simulink model "generate_joint_position_motion"  (R2023a)
settings: Solver=FixedStepDiscrete  StartTime=0.0  StopTime=inf  FixedStep=0.001  RelTol=1e-3  EnableMultiTasking=on
PreLoadFcn:
  | frs = FrankaRobotSettings;
libraries: franka_simulink_library x5
settings Model: SimulationMode=external  ExtModeTrigDuration=10000  Creator=vasi_ko  LastModifiedBy=kvasios
settings SolverCC: AlgebraicLoopSolver=TrustRegion
settings DataIOCC: LimitDataPoints=on  SaveFormat=Array  ReturnWorkspaceOutputs=off
settings OptimizationCC: DefaultParameterBehavior=Inlined  EnhancedBackFolding=on  PassReuseOutputArgsThreshold=0  OptimizeBlockOrder=speed  DifferentSizesBufferReuse=on  OptimizationCustomize=off
settings DebuggingCC: SolverPrmCheckMsg=warning  ParameterTunabilityLossMsg=error  UnconnectedInputMsg=warning  UnconnectedOutputMsg=warning  UnconnectedLineMsg=warning  SFUnexpectedBacktrackingDiag=warning  SFNoUnconditionalDefaultTransitionDiag=warning  SFExecutionAtInitializationDiag=none  ArithmeticOperatorsInVariantConditions=warning
settings ModelReferenceCC: EnableRefExpFcnMdlSchedulingChecks=on  PropagateSignalLabelsOutOfModel=off
settings SFSimCC: SimUseLocalCustomCode=off  MATLABDynamicMemAlloc=off  CustomCodeUndefinedFunction=UseInterfaceOnly  SimTargetLang=C++
settings RTWCC: RTWVerbose=off  RTWUseLocalCustomCode=off  BuildConfiguration=Faster Runs  TargetLang=C++  DLArmComputeVersion=19.05
settings CodeAppCC: ForceParamTrailComments=on  OperatorAnnotations=on
settings ConfigComp: CovMetricSettings=dw  CovSaveCumulativeToWorkspaceVar=on  CovSaveSingleToWorkspaceVar=on  CovExternalEMLEnable=off  CovSFcnEnable=off

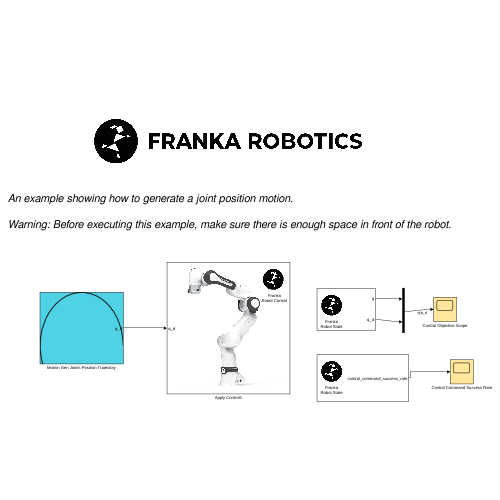
[thumbnail: Simulink's stored preview of the top-level diagram]
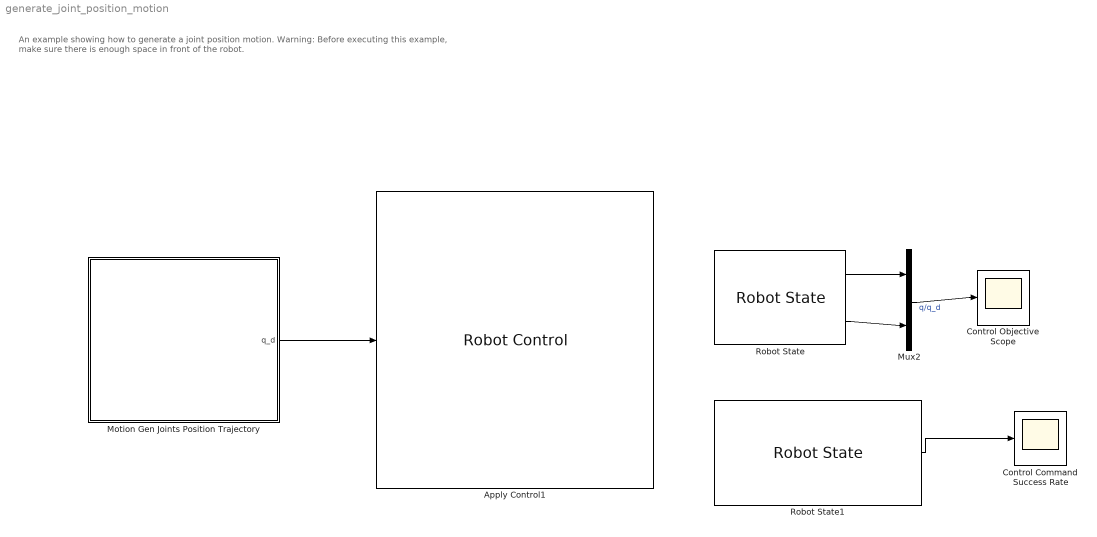
== system generate_joint_position_motion ==
  note: An example showing how to generate a joint position motion.
      |
      | Warning: Before executing this example, make sure there is enough space in front of the robot.
  Apply Control1 : franka_simulink_library/Robot Control  robot_ip=frs.robot_ip  gripper_selection=None  control_mode=Joint Positions - Internal Controller Mode  controller_choice=Joint Impedance Controller  joint_impedance=frs.joint_impedance_stiffness  cartesian_impedance=[3000, 3000, 3000, 300, 300, 300]  rate_limiter=on  cuttoff_frequency=frs.cutoff_frequency  elbow_control=off  collision_thresholds=frs.collision_thresholds.getAs1DArray  load_inertia=frs.load_inertia.getAs1DArray  NE_T_EE=frs.NE_T_EE(:)  EE_T_K=frs.EE_T_K(:)  init_joint_configuration_req=on  init_joint_configuration=frs.home_configuration
      settings: SourceProductName=Franka Robotics Simulink Support Package
  Control Command Success Rate : Scope
  Control Objective Scope : Scope
  Motion Gen Joints Position Trajectory : Subsystem
      mask Display:
      | pos = get_param(gcb, 'Position');
      | width = pos(3) - pos(1);
      | x = [0:width];
      | y = sin(x/180*pi);
      | % Parameters 'm' and 'b' must be defined in 'Parameters & Dialog' pane.
      | plot(cos(x/180*pi), sin(x/180*pi));
      | 
      | port_label('output',1,'q_d');
  Mux2 : Mux  Inputs=2
  Robot State : franka_simulink_library/Robot State  robot_ip=frs.robot_ip  signals_requested='q q_d'
      settings: SourceProductName=Franka Robotics Simulink Support Package
  Robot State1 : franka_simulink_library/Robot State  robot_ip=frs.robot_ip  signals_requested='control_command_success_rate'
      settings: SourceProductName=Franka Robotics Simulink Support Package
  wires:
  Robot State/2 -> Mux2/2
  Mux2/1 -> Control Objective Scope/1  "q/q_d"
  Motion Gen Joints Position Trajectory/1(q_d) -> Apply Control1/1
  Robot State/1 -> Mux2/1
  Robot State1/1 -> Control Command Success Rate/1

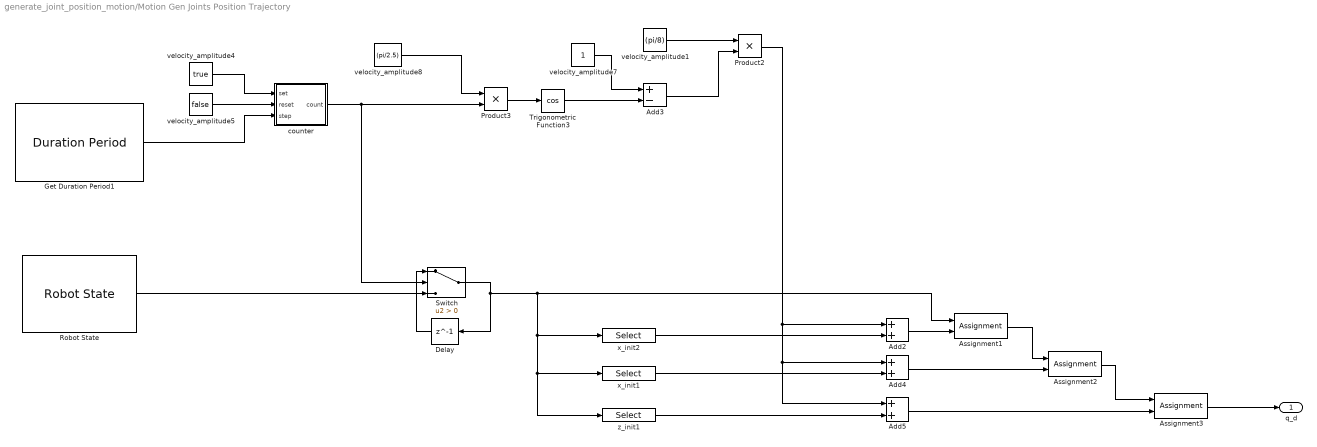
== system generate_joint_position_motion/Motion Gen Joints Position Trajectory ==
  Add2 : Sum
  Add3 : Sum  Inputs=+-
  Add4 : Sum
  Add5 : Sum
  Assignment1 : Assignment  DiagnosticForDimensions=Warning  IndexOptions=Index vector (dialog)  Indices=4  OutputSizes=1
  Assignment2 : Assignment  DiagnosticForDimensions=Warning  IndexOptions=Index vector (dialog)  Indices=5  OutputSizes=1
  Assignment3 : Assignment  DiagnosticForDimensions=Warning  IndexOptions=Index vector (dialog)  Indices=7  OutputSizes=1
  Delay : Delay  DelayLength=1
  Get Duration Period1 : franka_simulink_library/Duration Period  robot_ip=frs.robot_ip
      settings: SourceProductName=Franka Robotics Simulink Support Package
  Product2 : Product
  Product3 : Product
  Robot State : franka_simulink_library/Robot State  robot_ip=frs.robot_ip  signals_requested='q_d'
      settings: SourceProductName=Franka Robotics Simulink Support Package
  Switch : Switch  Criteria=u2 > Threshold  SaturateOnIntegerOverflow=off  InputSameDT=off
  Trigonometric Function3 : Trigonometry  Operator=cos
  counter : Subsystem
  velocity_amplitude1 : Constant  Value=(pi/8)  VectorParams1D=off
  velocity_amplitude4 : Constant  Value=true  VectorParams1D=off
  velocity_amplitude5 : Constant  Value=false  VectorParams1D=off
  velocity_amplitude7 : Constant  VectorParams1D=off
  velocity_amplitude8 : Constant  Value=(pi/2.5)  VectorParams1D=off
  x_init1 : Selector  InputPortWidth=7  IndexOptions=Index vector (dialog)  Indices=5  OutputSizes=1
  x_init2 : Selector  InputPortWidth=7  IndexOptions=Index vector (dialog)  Indices=4  OutputSizes=1
  z_init1 : Selector  InputPortWidth=7  IndexOptions=Index vector (dialog)  Indices=7  OutputSizes=1
  q_d : Outport  VectorParamsAs1DForOutWhenUnconnected=off
  wires:
  Add5/1 -> Assignment3/2
  Switch/1 -> Delay/1, z_init1/1, x_init1/1, x_init2/1, Assignment1/1
  Add4/1 -> Assignment2/2
  Assignment2/1 -> Assignment3/1
  z_init1/1 -> Add5/2
  x_init1/1 -> Add4/2
  Add2/1 -> Assignment1/2
  Assignment1/1 -> Assignment2/1
  x_init2/1 -> Add2/2
  velocity_amplitude1/1 -> Product2/1
  velocity_amplitude7/1 -> Add3/1
  Add3/1 -> Product2/2
  Product2/1 -> Add5/1, Add4/1, Add2/1
  Trigonometric Function3/1 -> Add3/2
  velocity_amplitude8/1 -> Product3/1
  Product3/1 -> Trigonometric Function3/1
  Assignment3/1 -> q_d/1
  Get Duration Period1/1 -> counter/3(step)
  velocity_amplitude4/1 -> counter/1(set)
  velocity_amplitude5/1 -> counter/2(reset)
  counter/1(count) -> Switch/2, Product3/2
  Delay/1 -> Switch/1
  Robot State/1 -> Switch/3

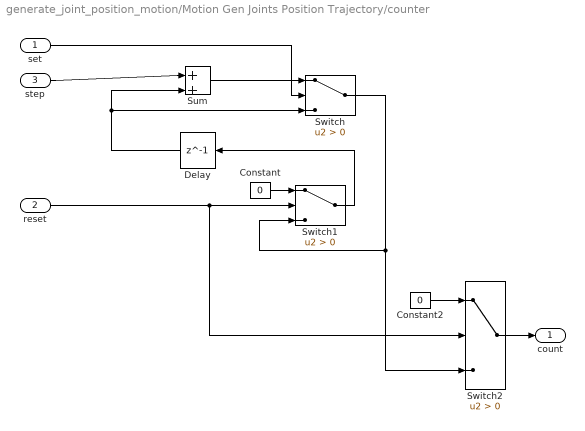
== system generate_joint_position_motion/Motion Gen Joints Position Trajectory/counter ==
  set : Inport  OutDataTypeStr=boolean
  reset : Inport  Port=2  OutDataTypeStr=boolean
  step : Inport  Port=3  OutDataTypeStr=double
  Constant : Constant  Value=0  OutDataTypeStr=double
  Constant2 : Constant  Value=0  OutDataTypeStr=double
  Delay : Delay  DelayLength=1  InitialCondition=0
  Sum : Sum  Inputs=|++
  Switch : Switch  Criteria=u2 > Threshold  SaturateOnIntegerOverflow=off  InputSameDT=off
  Switch1 : Switch  Criteria=u2 > Threshold  OutDataTypeStr=double  SaturateOnIntegerOverflow=off  InputSameDT=off
  Switch2 : Switch  Criteria=u2 > Threshold  OutDataTypeStr=double  SaturateOnIntegerOverflow=off  InputSameDT=off
  count : Outport  OutDataTypeStr=double  VectorParamsAs1DForOutWhenUnconnected=off
  wires:
  Switch2/1 -> count/1
  Constant2/1 -> Switch2/1
  Sum/1 -> Switch/1
  set/1 -> Switch/2
  Switch/1 -> Switch1/3, Switch2/3
  step/1 -> Sum/1
  Delay/1 -> Sum/2, Switch/3
  reset/1 -> Switch1/2, Switch2/2
  Constant/1 -> Switch1/1
  Switch1/1 -> Delay/1
